simulink model "SRLatchBlock"  (R2025a)
settings: Solver=VariableStepAuto  StartTime=0.0  StopTime=inf  RelTol=1e-3
settings Model: Creator=Soochan Kim  LastModifiedBy=Soochan Kim

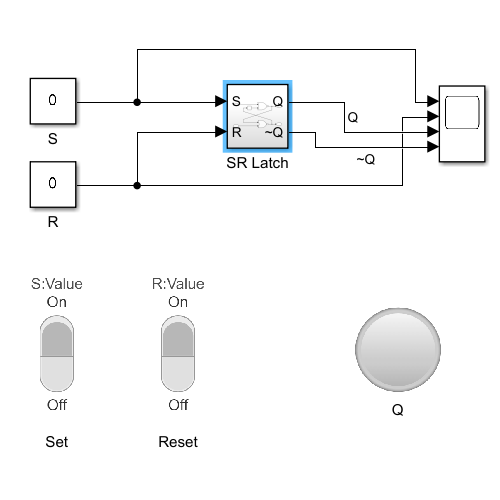
[thumbnail: Simulink's stored preview of the top-level diagram]
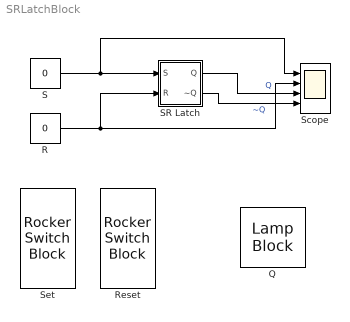
== system SRLatchBlock ==
  Q : LampBlock  LabelPosition=Hide  DefaultColor=[192.0, 192.0, 192.0]
  R : Constant  Value=0
  Reset : RockerSwitchBlock
  S : Constant  Value=0
  SR Latch : Subsystem
  Scope : Scope  NumInputPorts=4
      settings: ActiveDisplayYMinimum=-1  ActiveDisplayYMaximum=1
  Set : RockerSwitchBlock
  wires:
  S/1 -> Scope/1, SR Latch/1(S)
  R/1 -> Scope/2, SR Latch/2(R)
  SR Latch/1(Q) -> Scope/3  "Q"
  SR Latch/2(~Q) -> Scope/4  "~Q"

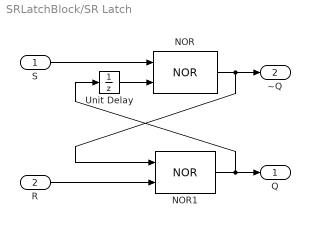
== system SRLatchBlock/SR Latch ==
  S : Inport
  R : Inport  Port=2
  NOR : Logic  Operator=NOR  IconShape=distinctive  AllPortsSameDT=off  OutDataTypeStr=boolean
  NOR1 : Logic  Operator=NOR  IconShape=distinctive  AllPortsSameDT=off  OutDataTypeStr=boolean
  Unit Delay : UnitDelay  SampleTime=-1  HasFrameUpgradeWarning=on
  Q : Outport
  ~Q : Outport  Port=2
  wires:
  NOR/1 -> ~Q/1, NOR1/1
  NOR1/1 -> Q/1, Unit Delay/1
  R/1 -> NOR1/2
  S/1 -> NOR/1
  Unit Delay/1 -> NOR/2
